simulink model "Bicopter_Dynamics"  (R2019a)
settings: Solver=ode4  StartTime=0.0  StopTime=5  FixedStep=0.001  RelTol=1e-3
undefined symbols (not defined in the file or in its folder): sigbuilder_block
settings Model: Creator=crsmyth  LastModifiedBy=Ross

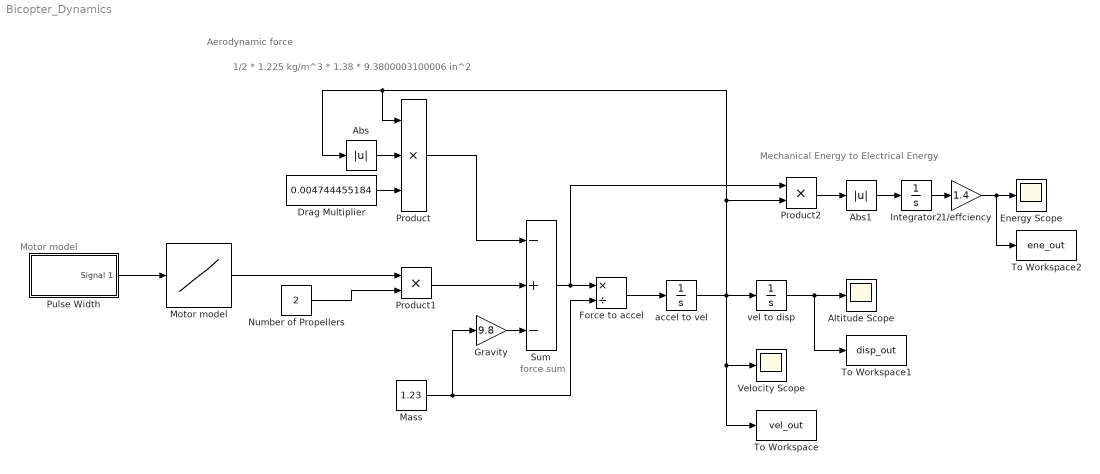
== system Bicopter_Dynamics ==
  note: force sum
  note: Motor model
  note: Aerodynamic force
  note: Mechanical Energy to Electrical Energy
  note: 1/2 * 1.225 kg/m^3 * 1.38 * 9.3800003100006 in^2
  1/effciency : Gain  Gain=1.4
  Abs : Abs
  Abs1 : Abs
  Altitude Scope : Scope
  Drag Multiplier : Constant  Value=0.004744455184
  Energy Scope : Scope
  Force to accel : Product  Inputs=*/
  Gravity : Gain  Gain=9.8
  Integrator2 : Integrator
  Mass : Constant  Value=1.23
  Motor model : Lookup_n-D  NumberOfTableDimensions=1  LookupTableObject=hi  BreakpointsForDimension1=[0,1,2]  Table=[0,0,9]  InternalRulePriority=Speed  RndMeth=Simplest  InputSameDT=on
  Number of Propellers : Constant  Value=2
  Product : Product  Inputs=3
  Product1 : Product
  Product2 : Product
  Pulse Width : Subsystem  Tag=STV Subsys  LoadFcn=sigbuilder_block('load');  StartFcn=sigbuilder_block('start');  StopFcn=sigbuilder_block('stop');  ClipboardFcn=sigbuilder_block('clipboard');  mask(Sigbuilder block){tuvar=[0:10]}
      mask help: Simulink:masks:SigbuilderBlock_MD
      mask init:
      | if ~strcmp(get_param(bdroot(gcbh),'SimulationStatus'),'stopped') tuvar = sigbuilder_block('maskInit'); end
      settings: CopyFcn=sigbuilder_block('copy');  DeleteFcn=sigbuilder_block('delete');  ModelCloseFcn=sigbuilder_block('modelClose');  PreSaveFcn=sigbuilder_block('preSave');  PauseFcn=sigbuilder_block('pause');  ContinueFcn=sigbuilder_block('continue');  NameChangeFcn=sigbuilder_block('namechange');  OpenFcn=sigbuilder_block('open',[480 108 550.8 360.6 ]);  CloseFcn=sigbuilder_block('close');
      mask Display: plot(0, 0, 100, 100,[2, 2, 32, 32, 2], [68, 8, 8, 68, 68],[32, 2], [38, 38], [32, 19, 2],[53, 60, 44], [32, 17, 17, 2],[16, 16, 31, 31]);txt = getActiveGroup(gcbh);text(2, 100, txt,'verticalAlignment', 'top');
  Sum : Sum  Inputs=-+-
  To Workspace : ToWorkspace  VariableName=vel_out  SampleTime=-1
      settings: Save2DSignal=2-D array (concatenate along first dimension)
  To Workspace1 : ToWorkspace  VariableName=disp_out  SampleTime=-1
      settings: Save2DSignal=2-D array (concatenate along first dimension)
  To Workspace2 : ToWorkspace  VariableName=ene_out  SampleTime=-1
      settings: Save2DSignal=2-D array (concatenate along first dimension)
  Velocity Scope : Scope
  accel to vel : Integrator
  vel to disp : Integrator
  wires:
  Sum/1 -> Force to accel/1, Product2/1
  Mass/1 -> Gravity/1, Force to accel/2
  Force to accel/1 -> accel to vel/1
  Gravity/1 -> Sum/3
  Product/1 -> Sum/1
  Drag Multiplier/1 -> Product/3
  Abs/1 -> Product/2
  Product1/1 -> Sum/2
  Number of Propellers/1 -> Product1/2
  Motor model/1 -> Product1/1
  1/effciency/1 -> To Workspace2/1, Energy Scope/1
  Pulse Width/1(Signal 1) -> Motor model/1
  accel to vel/1 -> vel to disp/1, Product2/2, Abs/1, Product/1, To Workspace/1, Velocity Scope/1
  Product2/1 -> Abs1/1
  Integrator2/1 -> 1/effciency/1
  Abs1/1 -> Integrator2/1
  vel to disp/1 -> To Workspace1/1, Altitude Scope/1

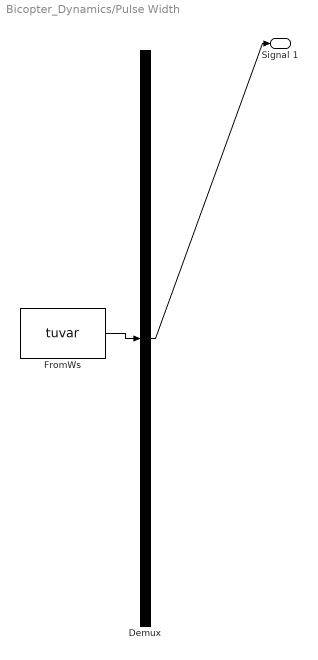
== system Bicopter_Dynamics/Pulse Width ==
  Demux : Demux  Tag=STV Demux  Outputs=1
  FromWs : FromWorkspace  Tag=STV FromWs  VariableName=tuvar  SampleTime=0
      SigBuilderData=|
      | common.afterFinalStr = 'Extrapolate'
      | common.sampleTime = 0
      | dataSet.timeRange = [0 5]
      | dataSet.name = 'Group 1'
      | sbobj.Groups.Name = 'Group 1'
      | sbobj.Groups.Signals.Name = 'Signal 1'
      | sbobj.Groups.Signals.XData = [0 0.646 0.646 0.9634 0.9634 5]
      | sbobj.Groups.Signals.YData = [2 2 1 1 1.66967 1.66967]
      | sbobj.Groups.TimeRange = [0 5]
  Signal 1 : Outport  Tag=STV Outport
  wires:
  FromWs/1 -> Demux/1
  Demux/1 -> Signal 1/1
